simulink model "FM_modulation (2)"  (R2023a)
settings: Solver=VariableStepAuto  StartTime=0.0  StopTime=.01  RelTol=1e-3
settings Model: Creator=USER  LastModifiedBy=USER

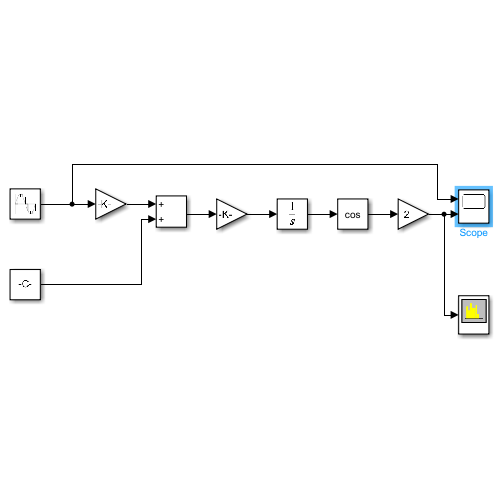
[thumbnail: Simulink's stored preview of the top-level diagram]
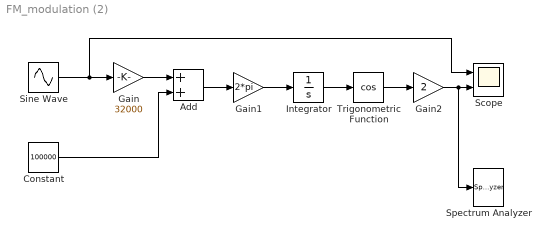
== system FM_modulation (2) ==
  Add : Sum
  Constant : Constant  Value=100000
  Gain : Gain  Gain=32000
  Gain1 : Gain  Gain=2*pi
  Gain2 : Gain  Gain=2
  Integrator : Integrator
  Scope : Scope  NumInputPorts=2
  Sine Wave : Sin  Amplitude=2  Frequency=2*pi*4000  SampleTime=0.000001
  Spectrum Analyzer : SpectrumAnalyzer  WindowPosition=[1.000000,49.000000,1536.000000,793.000000,]  ScopeFrameLocation=window  YLimits=[-45.76538668,20.88295305]  ColorLimits=[-80 20]  SelectedToolstripTab=spectrumAnalyzerToolstrip.spectrumTab
  Trigonometric Function : Trigonometry  Operator=cos
  wires:
  Gain/1 -> Add/1
  Integrator/1 -> Trigonometric Function/1
  Sine Wave/1 -> Scope/1, Gain/1
  Trigonometric Function/1 -> Gain2/1
  Gain2/1 -> Spectrum Analyzer/1, Scope/2
  Add/1 -> Gain1/1
  Constant/1 -> Add/2
  Gain1/1 -> Integrator/1
